simulink model "battery_pack_72v"  (R2020a)
settings: Solver=ode23t  StartTime=0.0  StopTime=5  RelTol=1e-3
libraries: fl_lib x1674, nesl_utility x2
(part 4 of 13)

== system battery_pack_72v/Battery_pack/Mod13/Cell2 ==
  Capacitor : fl_lib/Electrical/Electrical Elements/Capacitor  c=5000 F  r=1e-6 Ohm  g=0 1/Ohm  i_specify=off  i_priority=High  i=0 A  i_nominal_specify=off  i_nominal_unit=A  i_nominal_value=1  v_specify=off  v_priority=High  v=0 V  v_nominal_specify=off  v_nominal_unit=V  v_nominal_value=1  vc_specify=on  vc_priority=High  vc=0 V  vc_nominal_specify=off  vc_nominal_unit=V  vc_nominal_value=1
  DC Voltage Supply : fl_lib/Electrical/Electrical Sources/DC Voltage Source  v0=3.6 V
  Resistor1 : fl_lib/Electrical/Electrical Elements/Resistor  R=0.01 Ohm  i_specify=off  i_priority=High  i=0 A  i_nominal_specify=off  i_nominal_unit=A  i_nominal_value=1  v_specify=off  v_priority=High  v=0 V  v_nominal_specify=off  v_nominal_unit=V  v_nominal_value=1
  Resistor2 : fl_lib/Electrical/Electrical Elements/Resistor  R=0.005 Ohm  i_specify=off  i_priority=High  i=0 A  i_nominal_specify=off  i_nominal_unit=A  i_nominal_value=1  v_specify=off  v_priority=High  v=0 V  v_nominal_specify=off  v_nominal_unit=V  v_nominal_value=1
  + : PMIOPort  Side=Left
  - : PMIOPort  Port=2  Side=Right
  connections:
  DC Voltage Supply/LConn1 -- Resistor1/LConn1
  Capacitor/RConn1 -- +/RConn1 -- Resistor2/RConn1
  DC Voltage Supply/RConn1 -- -/RConn1
  Resistor1/RConn1 -- Capacitor/LConn1 -- Resistor2/LConn1

== system battery_pack_72v/Battery_pack/Mod13/Cell20 ==
  Capacitor : fl_lib/Electrical/Electrical Elements/Capacitor  c=5000 F  r=1e-6 Ohm  g=0 1/Ohm  i_specify=off  i_priority=High  i=0 A  i_nominal_specify=off  i_nominal_unit=A  i_nominal_value=1  v_specify=off  v_priority=High  v=0 V  v_nominal_specify=off  v_nominal_unit=V  v_nominal_value=1  vc_specify=on  vc_priority=High  vc=0 V  vc_nominal_specify=off  vc_nominal_unit=V  vc_nominal_value=1
  DC Voltage Supply : fl_lib/Electrical/Electrical Sources/DC Voltage Source  v0=3.6 V
  Resistor1 : fl_lib/Electrical/Electrical Elements/Resistor  R=0.01 Ohm  i_specify=off  i_priority=High  i=0 A  i_nominal_specify=off  i_nominal_unit=A  i_nominal_value=1  v_specify=off  v_priority=High  v=0 V  v_nominal_specify=off  v_nominal_unit=V  v_nominal_value=1
  Resistor2 : fl_lib/Electrical/Electrical Elements/Resistor  R=0.005 Ohm  i_specify=off  i_priority=High  i=0 A  i_nominal_specify=off  i_nominal_unit=A  i_nominal_value=1  v_specify=off  v_priority=High  v=0 V  v_nominal_specify=off  v_nominal_unit=V  v_nominal_value=1
  + : PMIOPort  Side=Left
  - : PMIOPort  Port=2  Side=Right
  connections:
  DC Voltage Supply/LConn1 -- Resistor1/LConn1
  Capacitor/RConn1 -- +/RConn1 -- Resistor2/RConn1
  DC Voltage Supply/RConn1 -- -/RConn1
  Resistor1/RConn1 -- Capacitor/LConn1 -- Resistor2/LConn1

== system battery_pack_72v/Battery_pack/Mod13/Cell21 ==
  Capacitor : fl_lib/Electrical/Electrical Elements/Capacitor  c=5000 F  r=1e-6 Ohm  g=0 1/Ohm  i_specify=off  i_priority=High  i=0 A  i_nominal_specify=off  i_nominal_unit=A  i_nominal_value=1  v_specify=off  v_priority=High  v=0 V  v_nominal_specify=off  v_nominal_unit=V  v_nominal_value=1  vc_specify=on  vc_priority=High  vc=0 V  vc_nominal_specify=off  vc_nominal_unit=V  vc_nominal_value=1
  DC Voltage Supply : fl_lib/Electrical/Electrical Sources/DC Voltage Source  v0=3.6 V
  Resistor1 : fl_lib/Electrical/Electrical Elements/Resistor  R=0.01 Ohm  i_specify=off  i_priority=High  i=0 A  i_nominal_specify=off  i_nominal_unit=A  i_nominal_value=1  v_specify=off  v_priority=High  v=0 V  v_nominal_specify=off  v_nominal_unit=V  v_nominal_value=1
  Resistor2 : fl_lib/Electrical/Electrical Elements/Resistor  R=0.005 Ohm  i_specify=off  i_priority=High  i=0 A  i_nominal_specify=off  i_nominal_unit=A  i_nominal_value=1  v_specify=off  v_priority=High  v=0 V  v_nominal_specify=off  v_nominal_unit=V  v_nominal_value=1
  + : PMIOPort  Side=Left
  - : PMIOPort  Port=2  Side=Right
  connections:
  Resistor2/LConn1 -- Capacitor/LConn1 -- Resistor1/RConn1
  DC Voltage Supply/RConn1 -- -/RConn1
  Resistor2/RConn1 -- +/RConn1 -- Capacitor/RConn1
  DC Voltage Supply/LConn1 -- Resistor1/LConn1

== system battery_pack_72v/Battery_pack/Mod13/Cell3 ==
  Capacitor : fl_lib/Electrical/Electrical Elements/Capacitor  c=5000 F  r=1e-6 Ohm  g=0 1/Ohm  i_specify=off  i_priority=High  i=0 A  i_nominal_specify=off  i_nominal_unit=A  i_nominal_value=1  v_specify=off  v_priority=High  v=0 V  v_nominal_specify=off  v_nominal_unit=V  v_nominal_value=1  vc_specify=on  vc_priority=High  vc=0 V  vc_nominal_specify=off  vc_nominal_unit=V  vc_nominal_value=1
  DC Voltage Supply : fl_lib/Electrical/Electrical Sources/DC Voltage Source  v0=3.6 V
  Resistor1 : fl_lib/Electrical/Electrical Elements/Resistor  R=0.01 Ohm  i_specify=off  i_priority=High  i=0 A  i_nominal_specify=off  i_nominal_unit=A  i_nominal_value=1  v_specify=off  v_priority=High  v=0 V  v_nominal_specify=off  v_nominal_unit=V  v_nominal_value=1
  Resistor2 : fl_lib/Electrical/Electrical Elements/Resistor  R=0.005 Ohm  i_specify=off  i_priority=High  i=0 A  i_nominal_specify=off  i_nominal_unit=A  i_nominal_value=1  v_specify=off  v_priority=High  v=0 V  v_nominal_specify=off  v_nominal_unit=V  v_nominal_value=1
  + : PMIOPort  Side=Left
  - : PMIOPort  Port=2  Side=Right
  connections:
  Resistor2/LConn1 -- Capacitor/LConn1 -- Resistor1/RConn1
  DC Voltage Supply/RConn1 -- -/RConn1
  Resistor2/RConn1 -- +/RConn1 -- Capacitor/RConn1
  DC Voltage Supply/LConn1 -- Resistor1/LConn1

== system battery_pack_72v/Battery_pack/Mod13/Cell4 ==
  Capacitor : fl_lib/Electrical/Electrical Elements/Capacitor  c=5000 F  r=1e-6 Ohm  g=0 1/Ohm  i_specify=off  i_priority=High  i=0 A  i_nominal_specify=off  i_nominal_unit=A  i_nominal_value=1  v_specify=off  v_priority=High  v=0 V  v_nominal_specify=off  v_nominal_unit=V  v_nominal_value=1  vc_specify=on  vc_priority=High  vc=0 V  vc_nominal_specify=off  vc_nominal_unit=V  vc_nominal_value=1
  DC Voltage Supply : fl_lib/Electrical/Electrical Sources/DC Voltage Source  v0=3.6 V
  Resistor1 : fl_lib/Electrical/Electrical Elements/Resistor  R=0.01 Ohm  i_specify=off  i_priority=High  i=0 A  i_nominal_specify=off  i_nominal_unit=A  i_nominal_value=1  v_specify=off  v_priority=High  v=0 V  v_nominal_specify=off  v_nominal_unit=V  v_nominal_value=1
  Resistor2 : fl_lib/Electrical/Electrical Elements/Resistor  R=0.005 Ohm  i_specify=off  i_priority=High  i=0 A  i_nominal_specify=off  i_nominal_unit=A  i_nominal_value=1  v_specify=off  v_priority=High  v=0 V  v_nominal_specify=off  v_nominal_unit=V  v_nominal_value=1
  + : PMIOPort  Side=Left
  - : PMIOPort  Port=2  Side=Right
  connections:
  DC Voltage Supply/LConn1 -- Resistor1/LConn1
  Capacitor/RConn1 -- +/RConn1 -- Resistor2/RConn1
  DC Voltage Supply/RConn1 -- -/RConn1
  Resistor1/RConn1 -- Capacitor/LConn1 -- Resistor2/LConn1

== system battery_pack_72v/Battery_pack/Mod13/Cell5 ==
  Capacitor : fl_lib/Electrical/Electrical Elements/Capacitor  c=5000 F  r=1e-6 Ohm  g=0 1/Ohm  i_specify=off  i_priority=High  i=0 A  i_nominal_specify=off  i_nominal_unit=A  i_nominal_value=1  v_specify=off  v_priority=High  v=0 V  v_nominal_specify=off  v_nominal_unit=V  v_nominal_value=1  vc_specify=on  vc_priority=High  vc=0 V  vc_nominal_specify=off  vc_nominal_unit=V  vc_nominal_value=1
  DC Voltage Supply : fl_lib/Electrical/Electrical Sources/DC Voltage Source  v0=3.6 V
  Resistor1 : fl_lib/Electrical/Electrical Elements/Resistor  R=0.01 Ohm  i_specify=off  i_priority=High  i=0 A  i_nominal_specify=off  i_nominal_unit=A  i_nominal_value=1  v_specify=off  v_priority=High  v=0 V  v_nominal_specify=off  v_nominal_unit=V  v_nominal_value=1
  Resistor2 : fl_lib/Electrical/Electrical Elements/Resistor  R=0.005 Ohm  i_specify=off  i_priority=High  i=0 A  i_nominal_specify=off  i_nominal_unit=A  i_nominal_value=1  v_specify=off  v_priority=High  v=0 V  v_nominal_specify=off  v_nominal_unit=V  v_nominal_value=1
  + : PMIOPort  Side=Left
  - : PMIOPort  Port=2  Side=Right
  connections:
  Resistor2/LConn1 -- Capacitor/LConn1 -- Resistor1/RConn1
  DC Voltage Supply/RConn1 -- -/RConn1
  Resistor2/RConn1 -- +/RConn1 -- Capacitor/RConn1
  DC Voltage Supply/LConn1 -- Resistor1/LConn1

== system battery_pack_72v/Battery_pack/Mod13/Cell6 ==
  Capacitor : fl_lib/Electrical/Electrical Elements/Capacitor  c=5000 F  r=1e-6 Ohm  g=0 1/Ohm  i_specify=off  i_priority=High  i=0 A  i_nominal_specify=off  i_nominal_unit=A  i_nominal_value=1  v_specify=off  v_priority=High  v=0 V  v_nominal_specify=off  v_nominal_unit=V  v_nominal_value=1  vc_specify=on  vc_priority=High  vc=0 V  vc_nominal_specify=off  vc_nominal_unit=V  vc_nominal_value=1
  DC Voltage Supply : fl_lib/Electrical/Electrical Sources/DC Voltage Source  v0=3.6 V
  Resistor1 : fl_lib/Electrical/Electrical Elements/Resistor  R=0.01 Ohm  i_specify=off  i_priority=High  i=0 A  i_nominal_specify=off  i_nominal_unit=A  i_nominal_value=1  v_specify=off  v_priority=High  v=0 V  v_nominal_specify=off  v_nominal_unit=V  v_nominal_value=1
  Resistor2 : fl_lib/Electrical/Electrical Elements/Resistor  R=0.005 Ohm  i_specify=off  i_priority=High  i=0 A  i_nominal_specify=off  i_nominal_unit=A  i_nominal_value=1  v_specify=off  v_priority=High  v=0 V  v_nominal_specify=off  v_nominal_unit=V  v_nominal_value=1
  + : PMIOPort  Side=Left
  - : PMIOPort  Port=2  Side=Right
  connections:
  DC Voltage Supply/LConn1 -- Resistor1/LConn1
  Capacitor/RConn1 -- +/RConn1 -- Resistor2/RConn1
  DC Voltage Supply/RConn1 -- -/RConn1
  Resistor1/RConn1 -- Capacitor/LConn1 -- Resistor2/LConn1

== system battery_pack_72v/Battery_pack/Mod13/Cell7 ==
  Capacitor : fl_lib/Electrical/Electrical Elements/Capacitor  c=5000 F  r=1e-6 Ohm  g=0 1/Ohm  i_specify=off  i_priority=High  i=0 A  i_nominal_specify=off  i_nominal_unit=A  i_nominal_value=1  v_specify=off  v_priority=High  v=0 V  v_nominal_specify=off  v_nominal_unit=V  v_nominal_value=1  vc_specify=on  vc_priority=High  vc=0 V  vc_nominal_specify=off  vc_nominal_unit=V  vc_nominal_value=1
  DC Voltage Supply : fl_lib/Electrical/Electrical Sources/DC Voltage Source  v0=3.6 V
  Resistor1 : fl_lib/Electrical/Electrical Elements/Resistor  R=0.01 Ohm  i_specify=off  i_priority=High  i=0 A  i_nominal_specify=off  i_nominal_unit=A  i_nominal_value=1  v_specify=off  v_priority=High  v=0 V  v_nominal_specify=off  v_nominal_unit=V  v_nominal_value=1
  Resistor2 : fl_lib/Electrical/Electrical Elements/Resistor  R=0.005 Ohm  i_specify=off  i_priority=High  i=0 A  i_nominal_specify=off  i_nominal_unit=A  i_nominal_value=1  v_specify=off  v_priority=High  v=0 V  v_nominal_specify=off  v_nominal_unit=V  v_nominal_value=1
  + : PMIOPort  Side=Left
  - : PMIOPort  Port=2  Side=Right
  connections:
  Resistor2/LConn1 -- Capacitor/LConn1 -- Resistor1/RConn1
  DC Voltage Supply/RConn1 -- -/RConn1
  Resistor2/RConn1 -- +/RConn1 -- Capacitor/RConn1
  DC Voltage Supply/LConn1 -- Resistor1/LConn1

== system battery_pack_72v/Battery_pack/Mod13/Cell8 ==
  Capacitor : fl_lib/Electrical/Electrical Elements/Capacitor  c=5000 F  r=1e-6 Ohm  g=0 1/Ohm  i_specify=off  i_priority=High  i=0 A  i_nominal_specify=off  i_nominal_unit=A  i_nominal_value=1  v_specify=off  v_priority=High  v=0 V  v_nominal_specify=off  v_nominal_unit=V  v_nominal_value=1  vc_specify=on  vc_priority=High  vc=0 V  vc_nominal_specify=off  vc_nominal_unit=V  vc_nominal_value=1
  DC Voltage Supply : fl_lib/Electrical/Electrical Sources/DC Voltage Source  v0=3.6 V
  Resistor1 : fl_lib/Electrical/Electrical Elements/Resistor  R=0.01 Ohm  i_specify=off  i_priority=High  i=0 A  i_nominal_specify=off  i_nominal_unit=A  i_nominal_value=1  v_specify=off  v_priority=High  v=0 V  v_nominal_specify=off  v_nominal_unit=V  v_nominal_value=1
  Resistor2 : fl_lib/Electrical/Electrical Elements/Resistor  R=0.005 Ohm  i_specify=off  i_priority=High  i=0 A  i_nominal_specify=off  i_nominal_unit=A  i_nominal_value=1  v_specify=off  v_priority=High  v=0 V  v_nominal_specify=off  v_nominal_unit=V  v_nominal_value=1
  + : PMIOPort  Side=Left
  - : PMIOPort  Port=2  Side=Right
  connections:
  DC Voltage Supply/LConn1 -- Resistor1/LConn1
  Capacitor/RConn1 -- +/RConn1 -- Resistor2/RConn1
  DC Voltage Supply/RConn1 -- -/RConn1
  Resistor1/RConn1 -- Capacitor/LConn1 -- Resistor2/LConn1

== system battery_pack_72v/Battery_pack/Mod13/Cell9 ==
  Capacitor : fl_lib/Electrical/Electrical Elements/Capacitor  c=5000 F  r=1e-6 Ohm  g=0 1/Ohm  i_specify=off  i_priority=High  i=0 A  i_nominal_specify=off  i_nominal_unit=A  i_nominal_value=1  v_specify=off  v_priority=High  v=0 V  v_nominal_specify=off  v_nominal_unit=V  v_nominal_value=1  vc_specify=on  vc_priority=High  vc=0 V  vc_nominal_specify=off  vc_nominal_unit=V  vc_nominal_value=1
  DC Voltage Supply : fl_lib/Electrical/Electrical Sources/DC Voltage Source  v0=3.6 V
  Resistor1 : fl_lib/Electrical/Electrical Elements/Resistor  R=0.01 Ohm  i_specify=off  i_priority=High  i=0 A  i_nominal_specify=off  i_nominal_unit=A  i_nominal_value=1  v_specify=off  v_priority=High  v=0 V  v_nominal_specify=off  v_nominal_unit=V  v_nominal_value=1
  Resistor2 : fl_lib/Electrical/Electrical Elements/Resistor  R=0.005 Ohm  i_specify=off  i_priority=High  i=0 A  i_nominal_specify=off  i_nominal_unit=A  i_nominal_value=1  v_specify=off  v_priority=High  v=0 V  v_nominal_specify=off  v_nominal_unit=V  v_nominal_value=1
  + : PMIOPort  Side=Left
  - : PMIOPort  Port=2  Side=Right
  connections:
  Resistor2/LConn1 -- Capacitor/LConn1 -- Resistor1/RConn1
  DC Voltage Supply/RConn1 -- -/RConn1
  Resistor2/RConn1 -- +/RConn1 -- Capacitor/RConn1
  DC Voltage Supply/LConn1 -- Resistor1/LConn1

== system battery_pack_72v/Battery_pack/Mod14/Cell1 ==
  Capacitor : fl_lib/Electrical/Electrical Elements/Capacitor  c=5000 F  r=1e-6 Ohm  g=0 1/Ohm  i_specify=off  i_priority=High  i=0 A  i_nominal_specify=off  i_nominal_unit=A  i_nominal_value=1  v_specify=off  v_priority=High  v=0 V  v_nominal_specify=off  v_nominal_unit=V  v_nominal_value=1  vc_specify=on  vc_priority=High  vc=0 V  vc_nominal_specify=off  vc_nominal_unit=V  vc_nominal_value=1
  DC Voltage Supply : fl_lib/Electrical/Electrical Sources/DC Voltage Source  v0=3.6 V
  Resistor1 : fl_lib/Electrical/Electrical Elements/Resistor  R=0.01 Ohm  i_specify=off  i_priority=High  i=0 A  i_nominal_specify=off  i_nominal_unit=A  i_nominal_value=1  v_specify=off  v_priority=High  v=0 V  v_nominal_specify=off  v_nominal_unit=V  v_nominal_value=1
  Resistor2 : fl_lib/Electrical/Electrical Elements/Resistor  R=0.005 Ohm  i_specify=off  i_priority=High  i=0 A  i_nominal_specify=off  i_nominal_unit=A  i_nominal_value=1  v_specify=off  v_priority=High  v=0 V  v_nominal_specify=off  v_nominal_unit=V  v_nominal_value=1
  + : PMIOPort  Side=Left
  - : PMIOPort  Port=2  Side=Right
  connections:
  DC Voltage Supply/LConn1 -- Resistor1/LConn1
  Capacitor/RConn1 -- +/RConn1 -- Resistor2/RConn1
  DC Voltage Supply/RConn1 -- -/RConn1
  Resistor1/RConn1 -- Capacitor/LConn1 -- Resistor2/LConn1

== system battery_pack_72v/Battery_pack/Mod14/Cell10 ==
  Capacitor : fl_lib/Electrical/Electrical Elements/Capacitor  c=5000 F  r=1e-6 Ohm  g=0 1/Ohm  i_specify=off  i_priority=High  i=0 A  i_nominal_specify=off  i_nominal_unit=A  i_nominal_value=1  v_specify=off  v_priority=High  v=0 V  v_nominal_specify=off  v_nominal_unit=V  v_nominal_value=1  vc_specify=on  vc_priority=High  vc=0 V  vc_nominal_specify=off  vc_nominal_unit=V  vc_nominal_value=1
  DC Voltage Supply : fl_lib/Electrical/Electrical Sources/DC Voltage Source  v0=3.6 V
  Resistor1 : fl_lib/Electrical/Electrical Elements/Resistor  R=0.01 Ohm  i_specify=off  i_priority=High  i=0 A  i_nominal_specify=off  i_nominal_unit=A  i_nominal_value=1  v_specify=off  v_priority=High  v=0 V  v_nominal_specify=off  v_nominal_unit=V  v_nominal_value=1
  Resistor2 : fl_lib/Electrical/Electrical Elements/Resistor  R=0.005 Ohm  i_specify=off  i_priority=High  i=0 A  i_nominal_specify=off  i_nominal_unit=A  i_nominal_value=1  v_specify=off  v_priority=High  v=0 V  v_nominal_specify=off  v_nominal_unit=V  v_nominal_value=1
  + : PMIOPort  Side=Left
  - : PMIOPort  Port=2  Side=Right
  connections:
  Resistor2/LConn1 -- Capacitor/LConn1 -- Resistor1/RConn1
  DC Voltage Supply/RConn1 -- -/RConn1
  Resistor2/RConn1 -- +/RConn1 -- Capacitor/RConn1
  DC Voltage Supply/LConn1 -- Resistor1/LConn1

== system battery_pack_72v/Battery_pack/Mod14/Cell11 ==
  Capacitor : fl_lib/Electrical/Electrical Elements/Capacitor  c=5000 F  r=1e-6 Ohm  g=0 1/Ohm  i_specify=off  i_priority=High  i=0 A  i_nominal_specify=off  i_nominal_unit=A  i_nominal_value=1  v_specify=off  v_priority=High  v=0 V  v_nominal_specify=off  v_nominal_unit=V  v_nominal_value=1  vc_specify=on  vc_priority=High  vc=0 V  vc_nominal_specify=off  vc_nominal_unit=V  vc_nominal_value=1
  DC Voltage Supply : fl_lib/Electrical/Electrical Sources/DC Voltage Source  v0=3.6 V
  Resistor1 : fl_lib/Electrical/Electrical Elements/Resistor  R=0.01 Ohm  i_specify=off  i_priority=High  i=0 A  i_nominal_specify=off  i_nominal_unit=A  i_nominal_value=1  v_specify=off  v_priority=High  v=0 V  v_nominal_specify=off  v_nominal_unit=V  v_nominal_value=1
  Resistor2 : fl_lib/Electrical/Electrical Elements/Resistor  R=0.005 Ohm  i_specify=off  i_priority=High  i=0 A  i_nominal_specify=off  i_nominal_unit=A  i_nominal_value=1  v_specify=off  v_priority=High  v=0 V  v_nominal_specify=off  v_nominal_unit=V  v_nominal_value=1
  + : PMIOPort  Side=Left
  - : PMIOPort  Port=2  Side=Right
  connections:
  DC Voltage Supply/LConn1 -- Resistor1/LConn1
  Capacitor/RConn1 -- +/RConn1 -- Resistor2/RConn1
  DC Voltage Supply/RConn1 -- -/RConn1
  Resistor1/RConn1 -- Capacitor/LConn1 -- Resistor2/LConn1

== system battery_pack_72v/Battery_pack/Mod14/Cell12 ==
  Capacitor : fl_lib/Electrical/Electrical Elements/Capacitor  c=5000 F  r=1e-6 Ohm  g=0 1/Ohm  i_specify=off  i_priority=High  i=0 A  i_nominal_specify=off  i_nominal_unit=A  i_nominal_value=1  v_specify=off  v_priority=High  v=0 V  v_nominal_specify=off  v_nominal_unit=V  v_nominal_value=1  vc_specify=on  vc_priority=High  vc=0 V  vc_nominal_specify=off  vc_nominal_unit=V  vc_nominal_value=1
  DC Voltage Supply : fl_lib/Electrical/Electrical Sources/DC Voltage Source  v0=3.6 V
  Resistor1 : fl_lib/Electrical/Electrical Elements/Resistor  R=0.01 Ohm  i_specify=off  i_priority=High  i=0 A  i_nominal_specify=off  i_nominal_unit=A  i_nominal_value=1  v_specify=off  v_priority=High  v=0 V  v_nominal_specify=off  v_nominal_unit=V  v_nominal_value=1
  Resistor2 : fl_lib/Electrical/Electrical Elements/Resistor  R=0.005 Ohm  i_specify=off  i_priority=High  i=0 A  i_nominal_specify=off  i_nominal_unit=A  i_nominal_value=1  v_specify=off  v_priority=High  v=0 V  v_nominal_specify=off  v_nominal_unit=V  v_nominal_value=1
  + : PMIOPort  Side=Left
  - : PMIOPort  Port=2  Side=Right
  connections:
  Resistor2/LConn1 -- Capacitor/LConn1 -- Resistor1/RConn1
  DC Voltage Supply/RConn1 -- -/RConn1
  Resistor2/RConn1 -- +/RConn1 -- Capacitor/RConn1
  DC Voltage Supply/LConn1 -- Resistor1/LConn1

== system battery_pack_72v/Battery_pack/Mod14/Cell15 ==
  Capacitor : fl_lib/Electrical/Electrical Elements/Capacitor  c=5000 F  r=1e-6 Ohm  g=0 1/Ohm  i_specify=off  i_priority=High  i=0 A  i_nominal_specify=off  i_nominal_unit=A  i_nominal_value=1  v_specify=off  v_priority=High  v=0 V  v_nominal_specify=off  v_nominal_unit=V  v_nominal_value=1  vc_specify=on  vc_priority=High  vc=0 V  vc_nominal_specify=off  vc_nominal_unit=V  vc_nominal_value=1
  DC Voltage Supply : fl_lib/Electrical/Electrical Sources/DC Voltage Source  v0=3.6 V
  Resistor1 : fl_lib/Electrical/Electrical Elements/Resistor  R=0.01 Ohm  i_specify=off  i_priority=High  i=0 A  i_nominal_specify=off  i_nominal_unit=A  i_nominal_value=1  v_specify=off  v_priority=High  v=0 V  v_nominal_specify=off  v_nominal_unit=V  v_nominal_value=1
  Resistor2 : fl_lib/Electrical/Electrical Elements/Resistor  R=0.005 Ohm  i_specify=off  i_priority=High  i=0 A  i_nominal_specify=off  i_nominal_unit=A  i_nominal_value=1  v_specify=off  v_priority=High  v=0 V  v_nominal_specify=off  v_nominal_unit=V  v_nominal_value=1
  + : PMIOPort  Side=Left
  - : PMIOPort  Port=2  Side=Right
  connections:
  DC Voltage Supply/LConn1 -- Resistor1/LConn1
  Capacitor/RConn1 -- +/RConn1 -- Resistor2/RConn1
  DC Voltage Supply/RConn1 -- -/RConn1
  Resistor1/RConn1 -- Capacitor/LConn1 -- Resistor2/LConn1

== system battery_pack_72v/Battery_pack/Mod14/Cell16 ==
  Capacitor : fl_lib/Electrical/Electrical Elements/Capacitor  c=5000 F  r=1e-6 Ohm  g=0 1/Ohm  i_specify=off  i_priority=High  i=0 A  i_nominal_specify=off  i_nominal_unit=A  i_nominal_value=1  v_specify=off  v_priority=High  v=0 V  v_nominal_specify=off  v_nominal_unit=V  v_nominal_value=1  vc_specify=on  vc_priority=High  vc=0 V  vc_nominal_specify=off  vc_nominal_unit=V  vc_nominal_value=1
  DC Voltage Supply : fl_lib/Electrical/Electrical Sources/DC Voltage Source  v0=3.6 V
  Resistor1 : fl_lib/Electrical/Electrical Elements/Resistor  R=0.01 Ohm  i_specify=off  i_priority=High  i=0 A  i_nominal_specify=off  i_nominal_unit=A  i_nominal_value=1  v_specify=off  v_priority=High  v=0 V  v_nominal_specify=off  v_nominal_unit=V  v_nominal_value=1
  Resistor2 : fl_lib/Electrical/Electrical Elements/Resistor  R=0.005 Ohm  i_specify=off  i_priority=High  i=0 A  i_nominal_specify=off  i_nominal_unit=A  i_nominal_value=1  v_specify=off  v_priority=High  v=0 V  v_nominal_specify=off  v_nominal_unit=V  v_nominal_value=1
  + : PMIOPort  Side=Left
  - : PMIOPort  Port=2  Side=Right
  connections:
  Resistor2/LConn1 -- Capacitor/LConn1 -- Resistor1/RConn1
  DC Voltage Supply/RConn1 -- -/RConn1
  Resistor2/RConn1 -- +/RConn1 -- Capacitor/RConn1
  DC Voltage Supply/LConn1 -- Resistor1/LConn1

== system battery_pack_72v/Battery_pack/Mod14/Cell17 ==
  Capacitor : fl_lib/Electrical/Electrical Elements/Capacitor  c=5000 F  r=1e-6 Ohm  g=0 1/Ohm  i_specify=off  i_priority=High  i=0 A  i_nominal_specify=off  i_nominal_unit=A  i_nominal_value=1  v_specify=off  v_priority=High  v=0 V  v_nominal_specify=off  v_nominal_unit=V  v_nominal_value=1  vc_specify=on  vc_priority=High  vc=0 V  vc_nominal_specify=off  vc_nominal_unit=V  vc_nominal_value=1
  DC Voltage Supply : fl_lib/Electrical/Electrical Sources/DC Voltage Source  v0=3.6 V
  Resistor1 : fl_lib/Electrical/Electrical Elements/Resistor  R=0.01 Ohm  i_specify=off  i_priority=High  i=0 A  i_nominal_specify=off  i_nominal_unit=A  i_nominal_value=1  v_specify=off  v_priority=High  v=0 V  v_nominal_specify=off  v_nominal_unit=V  v_nominal_value=1
  Resistor2 : fl_lib/Electrical/Electrical Elements/Resistor  R=0.005 Ohm  i_specify=off  i_priority=High  i=0 A  i_nominal_specify=off  i_nominal_unit=A  i_nominal_value=1  v_specify=off  v_priority=High  v=0 V  v_nominal_specify=off  v_nominal_unit=V  v_nominal_value=1
  + : PMIOPort  Side=Left
  - : PMIOPort  Port=2  Side=Right
  connections:
  DC Voltage Supply/LConn1 -- Resistor1/LConn1
  Capacitor/RConn1 -- +/RConn1 -- Resistor2/RConn1
  DC Voltage Supply/RConn1 -- -/RConn1
  Resistor1/RConn1 -- Capacitor/LConn1 -- Resistor2/LConn1

== system battery_pack_72v/Battery_pack/Mod14/Cell18 ==
  Capacitor : fl_lib/Electrical/Electrical Elements/Capacitor  c=5000 F  r=1e-6 Ohm  g=0 1/Ohm  i_specify=off  i_priority=High  i=0 A  i_nominal_specify=off  i_nominal_unit=A  i_nominal_value=1  v_specify=off  v_priority=High  v=0 V  v_nominal_specify=off  v_nominal_unit=V  v_nominal_value=1  vc_specify=on  vc_priority=High  vc=0 V  vc_nominal_specify=off  vc_nominal_unit=V  vc_nominal_value=1
  DC Voltage Supply : fl_lib/Electrical/Electrical Sources/DC Voltage Source  v0=3.6 V
  Resistor1 : fl_lib/Electrical/Electrical Elements/Resistor  R=0.01 Ohm  i_specify=off  i_priority=High  i=0 A  i_nominal_specify=off  i_nominal_unit=A  i_nominal_value=1  v_specify=off  v_priority=High  v=0 V  v_nominal_specify=off  v_nominal_unit=V  v_nominal_value=1
  Resistor2 : fl_lib/Electrical/Electrical Elements/Resistor  R=0.005 Ohm  i_specify=off  i_priority=High  i=0 A  i_nominal_specify=off  i_nominal_unit=A  i_nominal_value=1  v_specify=off  v_priority=High  v=0 V  v_nominal_specify=off  v_nominal_unit=V  v_nominal_value=1
  + : PMIOPort  Side=Left
  - : PMIOPort  Port=2  Side=Right
  connections:
  Resistor2/LConn1 -- Capacitor/LConn1 -- Resistor1/RConn1
  DC Voltage Supply/RConn1 -- -/RConn1
  Resistor2/RConn1 -- +/RConn1 -- Capacitor/RConn1
  DC Voltage Supply/LConn1 -- Resistor1/LConn1

== system battery_pack_72v/Battery_pack/Mod14/Cell19 ==
  Capacitor : fl_lib/Electrical/Electrical Elements/Capacitor  c=5000 F  r=1e-6 Ohm  g=0 1/Ohm  i_specify=off  i_priority=High  i=0 A  i_nominal_specify=off  i_nominal_unit=A  i_nominal_value=1  v_specify=off  v_priority=High  v=0 V  v_nominal_specify=off  v_nominal_unit=V  v_nominal_value=1  vc_specify=on  vc_priority=High  vc=0 V  vc_nominal_specify=off  vc_nominal_unit=V  vc_nominal_value=1
  DC Voltage Supply : fl_lib/Electrical/Electrical Sources/DC Voltage Source  v0=3.6 V
  Resistor1 : fl_lib/Electrical/Electrical Elements/Resistor  R=0.01 Ohm  i_specify=off  i_priority=High  i=0 A  i_nominal_specify=off  i_nominal_unit=A  i_nominal_value=1  v_specify=off  v_priority=High  v=0 V  v_nominal_specify=off  v_nominal_unit=V  v_nominal_value=1
  Resistor2 : fl_lib/Electrical/Electrical Elements/Resistor  R=0.005 Ohm  i_specify=off  i_priority=High  i=0 A  i_nominal_specify=off  i_nominal_unit=A  i_nominal_value=1  v_specify=off  v_priority=High  v=0 V  v_nominal_specify=off  v_nominal_unit=V  v_nominal_value=1
  + : PMIOPort  Side=Left
  - : PMIOPort  Port=2  Side=Right
  connections:
  DC Voltage Supply/LConn1 -- Resistor1/LConn1
  Capacitor/RConn1 -- +/RConn1 -- Resistor2/RConn1
  DC Voltage Supply/RConn1 -- -/RConn1
  Resistor1/RConn1 -- Capacitor/LConn1 -- Resistor2/LConn1

== system battery_pack_72v/Battery_pack/Mod14/Cell2 ==
  Capacitor : fl_lib/Electrical/Electrical Elements/Capacitor  c=5000 F  r=1e-6 Ohm  g=0 1/Ohm  i_specify=off  i_priority=High  i=0 A  i_nominal_specify=off  i_nominal_unit=A  i_nominal_value=1  v_specify=off  v_priority=High  v=0 V  v_nominal_specify=off  v_nominal_unit=V  v_nominal_value=1  vc_specify=on  vc_priority=High  vc=0 V  vc_nominal_specify=off  vc_nominal_unit=V  vc_nominal_value=1
  DC Voltage Supply : fl_lib/Electrical/Electrical Sources/DC Voltage Source  v0=3.6 V
  Resistor1 : fl_lib/Electrical/Electrical Elements/Resistor  R=0.01 Ohm  i_specify=off  i_priority=High  i=0 A  i_nominal_specify=off  i_nominal_unit=A  i_nominal_value=1  v_specify=off  v_priority=High  v=0 V  v_nominal_specify=off  v_nominal_unit=V  v_nominal_value=1
  Resistor2 : fl_lib/Electrical/Electrical Elements/Resistor  R=0.005 Ohm  i_specify=off  i_priority=High  i=0 A  i_nominal_specify=off  i_nominal_unit=A  i_nominal_value=1  v_specify=off  v_priority=High  v=0 V  v_nominal_specify=off  v_nominal_unit=V  v_nominal_value=1
  + : PMIOPort  Side=Left
  - : PMIOPort  Port=2  Side=Right
  connections:
  Resistor2/LConn1 -- Capacitor/LConn1 -- Resistor1/RConn1
  DC Voltage Supply/RConn1 -- -/RConn1
  Resistor2/RConn1 -- +/RConn1 -- Capacitor/RConn1
  DC Voltage Supply/LConn1 -- Resistor1/LConn1

== system battery_pack_72v/Battery_pack/Mod14/Cell20 ==
  Capacitor : fl_lib/Electrical/Electrical Elements/Capacitor  c=5000 F  r=1e-6 Ohm  g=0 1/Ohm  i_specify=off  i_priority=High  i=0 A  i_nominal_specify=off  i_nominal_unit=A  i_nominal_value=1  v_specify=off  v_priority=High  v=0 V  v_nominal_specify=off  v_nominal_unit=V  v_nominal_value=1  vc_specify=on  vc_priority=High  vc=0 V  vc_nominal_specify=off  vc_nominal_unit=V  vc_nominal_value=1
  DC Voltage Supply : fl_lib/Electrical/Electrical Sources/DC Voltage Source  v0=3.6 V
  Resistor1 : fl_lib/Electrical/Electrical Elements/Resistor  R=0.01 Ohm  i_specify=off  i_priority=High  i=0 A  i_nominal_specify=off  i_nominal_unit=A  i_nominal_value=1  v_specify=off  v_priority=High  v=0 V  v_nominal_specify=off  v_nominal_unit=V  v_nominal_value=1
  Resistor2 : fl_lib/Electrical/Electrical Elements/Resistor  R=0.005 Ohm  i_specify=off  i_priority=High  i=0 A  i_nominal_specify=off  i_nominal_unit=A  i_nominal_value=1  v_specify=off  v_priority=High  v=0 V  v_nominal_specify=off  v_nominal_unit=V  v_nominal_value=1
  + : PMIOPort  Side=Left
  - : PMIOPort  Port=2  Side=Right
  connections:
  Resistor2/LConn1 -- Capacitor/LConn1 -- Resistor1/RConn1
  DC Voltage Supply/RConn1 -- -/RConn1
  Resistor2/RConn1 -- +/RConn1 -- Capacitor/RConn1
  DC Voltage Supply/LConn1 -- Resistor1/LConn1

== system battery_pack_72v/Battery_pack/Mod14/Cell21 ==
  Capacitor : fl_lib/Electrical/Electrical Elements/Capacitor  c=5000 F  r=1e-6 Ohm  g=0 1/Ohm  i_specify=off  i_priority=High  i=0 A  i_nominal_specify=off  i_nominal_unit=A  i_nominal_value=1  v_specify=off  v_priority=High  v=0 V  v_nominal_specify=off  v_nominal_unit=V  v_nominal_value=1  vc_specify=on  vc_priority=High  vc=0 V  vc_nominal_specify=off  vc_nominal_unit=V  vc_nominal_value=1
  DC Voltage Supply : fl_lib/Electrical/Electrical Sources/DC Voltage Source  v0=3.6 V
  Resistor1 : fl_lib/Electrical/Electrical Elements/Resistor  R=0.01 Ohm  i_specify=off  i_priority=High  i=0 A  i_nominal_specify=off  i_nominal_unit=A  i_nominal_value=1  v_specify=off  v_priority=High  v=0 V  v_nominal_specify=off  v_nominal_unit=V  v_nominal_value=1
  Resistor2 : fl_lib/Electrical/Electrical Elements/Resistor  R=0.005 Ohm  i_specify=off  i_priority=High  i=0 A  i_nominal_specify=off  i_nominal_unit=A  i_nominal_value=1  v_specify=off  v_priority=High  v=0 V  v_nominal_specify=off  v_nominal_unit=V  v_nominal_value=1
  + : PMIOPort  Side=Left
  - : PMIOPort  Port=2  Side=Right
  connections:
  DC Voltage Supply/LConn1 -- Resistor1/LConn1
  Capacitor/RConn1 -- +/RConn1 -- Resistor2/RConn1
  DC Voltage Supply/RConn1 -- -/RConn1
  Resistor1/RConn1 -- Capacitor/LConn1 -- Resistor2/LConn1

== system battery_pack_72v/Battery_pack/Mod14/Cell3 ==
  Capacitor : fl_lib/Electrical/Electrical Elements/Capacitor  c=5000 F  r=1e-6 Ohm  g=0 1/Ohm  i_specify=off  i_priority=High  i=0 A  i_nominal_specify=off  i_nominal_unit=A  i_nominal_value=1  v_specify=off  v_priority=High  v=0 V  v_nominal_specify=off  v_nominal_unit=V  v_nominal_value=1  vc_specify=on  vc_priority=High  vc=0 V  vc_nominal_specify=off  vc_nominal_unit=V  vc_nominal_value=1
  DC Voltage Supply : fl_lib/Electrical/Electrical Sources/DC Voltage Source  v0=3.6 V
  Resistor1 : fl_lib/Electrical/Electrical Elements/Resistor  R=0.01 Ohm  i_specify=off  i_priority=High  i=0 A  i_nominal_specify=off  i_nominal_unit=A  i_nominal_value=1  v_specify=off  v_priority=High  v=0 V  v_nominal_specify=off  v_nominal_unit=V  v_nominal_value=1
  Resistor2 : fl_lib/Electrical/Electrical Elements/Resistor  R=0.005 Ohm  i_specify=off  i_priority=High  i=0 A  i_nominal_specify=off  i_nominal_unit=A  i_nominal_value=1  v_specify=off  v_priority=High  v=0 V  v_nominal_specify=off  v_nominal_unit=V  v_nominal_value=1
  + : PMIOPort  Side=Left
  - : PMIOPort  Port=2  Side=Right
  connections:
  DC Voltage Supply/LConn1 -- Resistor1/LConn1
  Capacitor/RConn1 -- +/RConn1 -- Resistor2/RConn1
  DC Voltage Supply/RConn1 -- -/RConn1
  Resistor1/RConn1 -- Capacitor/LConn1 -- Resistor2/LConn1

== system battery_pack_72v/Battery_pack/Mod14/Cell4 ==
  Capacitor : fl_lib/Electrical/Electrical Elements/Capacitor  c=5000 F  r=1e-6 Ohm  g=0 1/Ohm  i_specify=off  i_priority=High  i=0 A  i_nominal_specify=off  i_nominal_unit=A  i_nominal_value=1  v_specify=off  v_priority=High  v=0 V  v_nominal_specify=off  v_nominal_unit=V  v_nominal_value=1  vc_specify=on  vc_priority=High  vc=0 V  vc_nominal_specify=off  vc_nominal_unit=V  vc_nominal_value=1
  DC Voltage Supply : fl_lib/Electrical/Electrical Sources/DC Voltage Source  v0=3.6 V
  Resistor1 : fl_lib/Electrical/Electrical Elements/Resistor  R=0.01 Ohm  i_specify=off  i_priority=High  i=0 A  i_nominal_specify=off  i_nominal_unit=A  i_nominal_value=1  v_specify=off  v_priority=High  v=0 V  v_nominal_specify=off  v_nominal_unit=V  v_nominal_value=1
  Resistor2 : fl_lib/Electrical/Electrical Elements/Resistor  R=0.005 Ohm  i_specify=off  i_priority=High  i=0 A  i_nominal_specify=off  i_nominal_unit=A  i_nominal_value=1  v_specify=off  v_priority=High  v=0 V  v_nominal_specify=off  v_nominal_unit=V  v_nominal_value=1
  + : PMIOPort  Side=Left
  - : PMIOPort  Port=2  Side=Right
  connections:
  Resistor2/LConn1 -- Capacitor/LConn1 -- Resistor1/RConn1
  DC Voltage Supply/RConn1 -- -/RConn1
  Resistor2/RConn1 -- +/RConn1 -- Capacitor/RConn1
  DC Voltage Supply/LConn1 -- Resistor1/LConn1

== system battery_pack_72v/Battery_pack/Mod14/Cell5 ==
  Capacitor : fl_lib/Electrical/Electrical Elements/Capacitor  c=5000 F  r=1e-6 Ohm  g=0 1/Ohm  i_specify=off  i_priority=High  i=0 A  i_nominal_specify=off  i_nominal_unit=A  i_nominal_value=1  v_specify=off  v_priority=High  v=0 V  v_nominal_specify=off  v_nominal_unit=V  v_nominal_value=1  vc_specify=on  vc_priority=High  vc=0 V  vc_nominal_specify=off  vc_nominal_unit=V  vc_nominal_value=1
  DC Voltage Supply : fl_lib/Electrical/Electrical Sources/DC Voltage Source  v0=3.6 V
  Resistor1 : fl_lib/Electrical/Electrical Elements/Resistor  R=0.01 Ohm  i_specify=off  i_priority=High  i=0 A  i_nominal_specify=off  i_nominal_unit=A  i_nominal_value=1  v_specify=off  v_priority=High  v=0 V  v_nominal_specify=off  v_nominal_unit=V  v_nominal_value=1
  Resistor2 : fl_lib/Electrical/Electrical Elements/Resistor  R=0.005 Ohm  i_specify=off  i_priority=High  i=0 A  i_nominal_specify=off  i_nominal_unit=A  i_nominal_value=1  v_specify=off  v_priority=High  v=0 V  v_nominal_specify=off  v_nominal_unit=V  v_nominal_value=1
  + : PMIOPort  Side=Left
  - : PMIOPort  Port=2  Side=Right
  connections:
  DC Voltage Supply/LConn1 -- Resistor1/LConn1
  Capacitor/RConn1 -- +/RConn1 -- Resistor2/RConn1
  DC Voltage Supply/RConn1 -- -/RConn1
  Resistor1/RConn1 -- Capacitor/LConn1 -- Resistor2/LConn1

== system battery_pack_72v/Battery_pack/Mod14/Cell6 ==
  Capacitor : fl_lib/Electrical/Electrical Elements/Capacitor  c=5000 F  r=1e-6 Ohm  g=0 1/Ohm  i_specify=off  i_priority=High  i=0 A  i_nominal_specify=off  i_nominal_unit=A  i_nominal_value=1  v_specify=off  v_priority=High  v=0 V  v_nominal_specify=off  v_nominal_unit=V  v_nominal_value=1  vc_specify=on  vc_priority=High  vc=0 V  vc_nominal_specify=off  vc_nominal_unit=V  vc_nominal_value=1
  DC Voltage Supply : fl_lib/Electrical/Electrical Sources/DC Voltage Source  v0=3.6 V
  Resistor1 : fl_lib/Electrical/Electrical Elements/Resistor  R=0.01 Ohm  i_specify=off  i_priority=High  i=0 A  i_nominal_specify=off  i_nominal_unit=A  i_nominal_value=1  v_specify=off  v_priority=High  v=0 V  v_nominal_specify=off  v_nominal_unit=V  v_nominal_value=1
  Resistor2 : fl_lib/Electrical/Electrical Elements/Resistor  R=0.005 Ohm  i_specify=off  i_priority=High  i=0 A  i_nominal_specify=off  i_nominal_unit=A  i_nominal_value=1  v_specify=off  v_priority=High  v=0 V  v_nominal_specify=off  v_nominal_unit=V  v_nominal_value=1
  + : PMIOPort  Side=Left
  - : PMIOPort  Port=2  Side=Right
  connections:
  Resistor2/LConn1 -- Capacitor/LConn1 -- Resistor1/RConn1
  DC Voltage Supply/RConn1 -- -/RConn1
  Resistor2/RConn1 -- +/RConn1 -- Capacitor/RConn1
  DC Voltage Supply/LConn1 -- Resistor1/LConn1

== system battery_pack_72v/Battery_pack/Mod14/Cell7 ==
  Capacitor : fl_lib/Electrical/Electrical Elements/Capacitor  c=5000 F  r=1e-6 Ohm  g=0 1/Ohm  i_specify=off  i_priority=High  i=0 A  i_nominal_specify=off  i_nominal_unit=A  i_nominal_value=1  v_specify=off  v_priority=High  v=0 V  v_nominal_specify=off  v_nominal_unit=V  v_nominal_value=1  vc_specify=on  vc_priority=High  vc=0 V  vc_nominal_specify=off  vc_nominal_unit=V  vc_nominal_value=1
  DC Voltage Supply : fl_lib/Electrical/Electrical Sources/DC Voltage Source  v0=3.6 V
  Resistor1 : fl_lib/Electrical/Electrical Elements/Resistor  R=0.01 Ohm  i_specify=off  i_priority=High  i=0 A  i_nominal_specify=off  i_nominal_unit=A  i_nominal_value=1  v_specify=off  v_priority=High  v=0 V  v_nominal_specify=off  v_nominal_unit=V  v_nominal_value=1
  Resistor2 : fl_lib/Electrical/Electrical Elements/Resistor  R=0.005 Ohm  i_specify=off  i_priority=High  i=0 A  i_nominal_specify=off  i_nominal_unit=A  i_nominal_value=1  v_specify=off  v_priority=High  v=0 V  v_nominal_specify=off  v_nominal_unit=V  v_nominal_value=1
  + : PMIOPort  Side=Left
  - : PMIOPort  Port=2  Side=Right
  connections:
  DC Voltage Supply/LConn1 -- Resistor1/LConn1
  Capacitor/RConn1 -- +/RConn1 -- Resistor2/RConn1
  DC Voltage Supply/RConn1 -- -/RConn1
  Resistor1/RConn1 -- Capacitor/LConn1 -- Resistor2/LConn1

== system battery_pack_72v/Battery_pack/Mod14/Cell8 ==
  Capacitor : fl_lib/Electrical/Electrical Elements/Capacitor  c=5000 F  r=1e-6 Ohm  g=0 1/Ohm  i_specify=off  i_priority=High  i=0 A  i_nominal_specify=off  i_nominal_unit=A  i_nominal_value=1  v_specify=off  v_priority=High  v=0 V  v_nominal_specify=off  v_nominal_unit=V  v_nominal_value=1  vc_specify=on  vc_priority=High  vc=0 V  vc_nominal_specify=off  vc_nominal_unit=V  vc_nominal_value=1
  DC Voltage Supply : fl_lib/Electrical/Electrical Sources/DC Voltage Source  v0=3.6 V
  Resistor1 : fl_lib/Electrical/Electrical Elements/Resistor  R=0.01 Ohm  i_specify=off  i_priority=High  i=0 A  i_nominal_specify=off  i_nominal_unit=A  i_nominal_value=1  v_specify=off  v_priority=High  v=0 V  v_nominal_specify=off  v_nominal_unit=V  v_nominal_value=1
  Resistor2 : fl_lib/Electrical/Electrical Elements/Resistor  R=0.005 Ohm  i_specify=off  i_priority=High  i=0 A  i_nominal_specify=off  i_nominal_unit=A  i_nominal_value=1  v_specify=off  v_priority=High  v=0 V  v_nominal_specify=off  v_nominal_unit=V  v_nominal_value=1
  + : PMIOPort  Side=Left
  - : PMIOPort  Port=2  Side=Right
  connections:
  Resistor2/LConn1 -- Capacitor/LConn1 -- Resistor1/RConn1
  DC Voltage Supply/RConn1 -- -/RConn1
  Resistor2/RConn1 -- +/RConn1 -- Capacitor/RConn1
  DC Voltage Supply/LConn1 -- Resistor1/LConn1

== system battery_pack_72v/Battery_pack/Mod14/Cell9 ==
  Capacitor : fl_lib/Electrical/Electrical Elements/Capacitor  c=5000 F  r=1e-6 Ohm  g=0 1/Ohm  i_specify=off  i_priority=High  i=0 A  i_nominal_specify=off  i_nominal_unit=A  i_nominal_value=1  v_specify=off  v_priority=High  v=0 V  v_nominal_specify=off  v_nominal_unit=V  v_nominal_value=1  vc_specify=on  vc_priority=High  vc=0 V  vc_nominal_specify=off  vc_nominal_unit=V  vc_nominal_value=1
  DC Voltage Supply : fl_lib/Electrical/Electrical Sources/DC Voltage Source  v0=3.6 V
  Resistor1 : fl_lib/Electrical/Electrical Elements/Resistor  R=0.01 Ohm  i_specify=off  i_priority=High  i=0 A  i_nominal_specify=off  i_nominal_unit=A  i_nominal_value=1  v_specify=off  v_priority=High  v=0 V  v_nominal_specify=off  v_nominal_unit=V  v_nominal_value=1
  Resistor2 : fl_lib/Electrical/Electrical Elements/Resistor  R=0.005 Ohm  i_specify=off  i_priority=High  i=0 A  i_nominal_specify=off  i_nominal_unit=A  i_nominal_value=1  v_specify=off  v_priority=High  v=0 V  v_nominal_specify=off  v_nominal_unit=V  v_nominal_value=1
  + : PMIOPort  Side=Left
  - : PMIOPort  Port=2  Side=Right
  connections:
  DC Voltage Supply/LConn1 -- Resistor1/LConn1
  Capacitor/RConn1 -- +/RConn1 -- Resistor2/RConn1
  DC Voltage Supply/RConn1 -- -/RConn1
  Resistor1/RConn1 -- Capacitor/LConn1 -- Resistor2/LConn1

== system battery_pack_72v/Battery_pack/Mod15/Cell1 ==
  Capacitor : fl_lib/Electrical/Electrical Elements/Capacitor  c=5000 F  r=1e-6 Ohm  g=0 1/Ohm  i_specify=off  i_priority=High  i=0 A  i_nominal_specify=off  i_nominal_unit=A  i_nominal_value=1  v_specify=off  v_priority=High  v=0 V  v_nominal_specify=off  v_nominal_unit=V  v_nominal_value=1  vc_specify=on  vc_priority=High  vc=0 V  vc_nominal_specify=off  vc_nominal_unit=V  vc_nominal_value=1
  DC Voltage Supply : fl_lib/Electrical/Electrical Sources/DC Voltage Source  v0=3.6 V
  Resistor1 : fl_lib/Electrical/Electrical Elements/Resistor  R=0.01 Ohm  i_specify=off  i_priority=High  i=0 A  i_nominal_specify=off  i_nominal_unit=A  i_nominal_value=1  v_specify=off  v_priority=High  v=0 V  v_nominal_specify=off  v_nominal_unit=V  v_nominal_value=1
  Resistor2 : fl_lib/Electrical/Electrical Elements/Resistor  R=0.005 Ohm  i_specify=off  i_priority=High  i=0 A  i_nominal_specify=off  i_nominal_unit=A  i_nominal_value=1  v_specify=off  v_priority=High  v=0 V  v_nominal_specify=off  v_nominal_unit=V  v_nominal_value=1
  + : PMIOPort  Side=Left
  - : PMIOPort  Port=2  Side=Right
  connections:
  Resistor2/LConn1 -- Capacitor/LConn1 -- Resistor1/RConn1
  DC Voltage Supply/RConn1 -- -/RConn1
  Resistor2/RConn1 -- +/RConn1 -- Capacitor/RConn1
  DC Voltage Supply/LConn1 -- Resistor1/LConn1

== system battery_pack_72v/Battery_pack/Mod15/Cell10 ==
  Capacitor : fl_lib/Electrical/Electrical Elements/Capacitor  c=5000 F  r=1e-6 Ohm  g=0 1/Ohm  i_specify=off  i_priority=High  i=0 A  i_nominal_specify=off  i_nominal_unit=A  i_nominal_value=1  v_specify=off  v_priority=High  v=0 V  v_nominal_specify=off  v_nominal_unit=V  v_nominal_value=1  vc_specify=on  vc_priority=High  vc=0 V  vc_nominal_specify=off  vc_nominal_unit=V  vc_nominal_value=1
  DC Voltage Supply : fl_lib/Electrical/Electrical Sources/DC Voltage Source  v0=3.6 V
  Resistor1 : fl_lib/Electrical/Electrical Elements/Resistor  R=0.01 Ohm  i_specify=off  i_priority=High  i=0 A  i_nominal_specify=off  i_nominal_unit=A  i_nominal_value=1  v_specify=off  v_priority=High  v=0 V  v_nominal_specify=off  v_nominal_unit=V  v_nominal_value=1
  Resistor2 : fl_lib/Electrical/Electrical Elements/Resistor  R=0.005 Ohm  i_specify=off  i_priority=High  i=0 A  i_nominal_specify=off  i_nominal_unit=A  i_nominal_value=1  v_specify=off  v_priority=High  v=0 V  v_nominal_specify=off  v_nominal_unit=V  v_nominal_value=1
  + : PMIOPort  Side=Left
  - : PMIOPort  Port=2  Side=Right
  connections:
  DC Voltage Supply/LConn1 -- Resistor1/LConn1
  Capacitor/RConn1 -- +/RConn1 -- Resistor2/RConn1
  DC Voltage Supply/RConn1 -- -/RConn1
  Resistor1/RConn1 -- Capacitor/LConn1 -- Resistor2/LConn1

== system battery_pack_72v/Battery_pack/Mod15/Cell11 ==
  Capacitor : fl_lib/Electrical/Electrical Elements/Capacitor  c=5000 F  r=1e-6 Ohm  g=0 1/Ohm  i_specify=off  i_priority=High  i=0 A  i_nominal_specify=off  i_nominal_unit=A  i_nominal_value=1  v_specify=off  v_priority=High  v=0 V  v_nominal_specify=off  v_nominal_unit=V  v_nominal_value=1  vc_specify=on  vc_priority=High  vc=0 V  vc_nominal_specify=off  vc_nominal_unit=V  vc_nominal_value=1
  DC Voltage Supply : fl_lib/Electrical/Electrical Sources/DC Voltage Source  v0=3.6 V
  Resistor1 : fl_lib/Electrical/Electrical Elements/Resistor  R=0.01 Ohm  i_specify=off  i_priority=High  i=0 A  i_nominal_specify=off  i_nominal_unit=A  i_nominal_value=1  v_specify=off  v_priority=High  v=0 V  v_nominal_specify=off  v_nominal_unit=V  v_nominal_value=1
  Resistor2 : fl_lib/Electrical/Electrical Elements/Resistor  R=0.005 Ohm  i_specify=off  i_priority=High  i=0 A  i_nominal_specify=off  i_nominal_unit=A  i_nominal_value=1  v_specify=off  v_priority=High  v=0 V  v_nominal_specify=off  v_nominal_unit=V  v_nominal_value=1
  + : PMIOPort  Side=Left
  - : PMIOPort  Port=2  Side=Right
  connections:
  Resistor2/LConn1 -- Capacitor/LConn1 -- Resistor1/RConn1
  DC Voltage Supply/RConn1 -- -/RConn1
  Resistor2/RConn1 -- +/RConn1 -- Capacitor/RConn1
  DC Voltage Supply/LConn1 -- Resistor1/LConn1

== system battery_pack_72v/Battery_pack/Mod15/Cell12 ==
  Capacitor : fl_lib/Electrical/Electrical Elements/Capacitor  c=5000 F  r=1e-6 Ohm  g=0 1/Ohm  i_specify=off  i_priority=High  i=0 A  i_nominal_specify=off  i_nominal_unit=A  i_nominal_value=1  v_specify=off  v_priority=High  v=0 V  v_nominal_specify=off  v_nominal_unit=V  v_nominal_value=1  vc_specify=on  vc_priority=High  vc=0 V  vc_nominal_specify=off  vc_nominal_unit=V  vc_nominal_value=1
  DC Voltage Supply : fl_lib/Electrical/Electrical Sources/DC Voltage Source  v0=3.6 V
  Resistor1 : fl_lib/Electrical/Electrical Elements/Resistor  R=0.01 Ohm  i_specify=off  i_priority=High  i=0 A  i_nominal_specify=off  i_nominal_unit=A  i_nominal_value=1  v_specify=off  v_priority=High  v=0 V  v_nominal_specify=off  v_nominal_unit=V  v_nominal_value=1
  Resistor2 : fl_lib/Electrical/Electrical Elements/Resistor  R=0.005 Ohm  i_specify=off  i_priority=High  i=0 A  i_nominal_specify=off  i_nominal_unit=A  i_nominal_value=1  v_specify=off  v_priority=High  v=0 V  v_nominal_specify=off  v_nominal_unit=V  v_nominal_value=1
  + : PMIOPort  Side=Left
  - : PMIOPort  Port=2  Side=Right
  connections:
  DC Voltage Supply/LConn1 -- Resistor1/LConn1
  Capacitor/RConn1 -- +/RConn1 -- Resistor2/RConn1
  DC Voltage Supply/RConn1 -- -/RConn1
  Resistor1/RConn1 -- Capacitor/LConn1 -- Resistor2/LConn1

== system battery_pack_72v/Battery_pack/Mod15/Cell15 ==
  Capacitor : fl_lib/Electrical/Electrical Elements/Capacitor  c=5000 F  r=1e-6 Ohm  g=0 1/Ohm  i_specify=off  i_priority=High  i=0 A  i_nominal_specify=off  i_nominal_unit=A  i_nominal_value=1  v_specify=off  v_priority=High  v=0 V  v_nominal_specify=off  v_nominal_unit=V  v_nominal_value=1  vc_specify=on  vc_priority=High  vc=0 V  vc_nominal_specify=off  vc_nominal_unit=V  vc_nominal_value=1
  DC Voltage Supply : fl_lib/Electrical/Electrical Sources/DC Voltage Source  v0=3.6 V
  Resistor1 : fl_lib/Electrical/Electrical Elements/Resistor  R=0.01 Ohm  i_specify=off  i_priority=High  i=0 A  i_nominal_specify=off  i_nominal_unit=A  i_nominal_value=1  v_specify=off  v_priority=High  v=0 V  v_nominal_specify=off  v_nominal_unit=V  v_nominal_value=1
  Resistor2 : fl_lib/Electrical/Electrical Elements/Resistor  R=0.005 Ohm  i_specify=off  i_priority=High  i=0 A  i_nominal_specify=off  i_nominal_unit=A  i_nominal_value=1  v_specify=off  v_priority=High  v=0 V  v_nominal_specify=off  v_nominal_unit=V  v_nominal_value=1
  + : PMIOPort  Side=Left
  - : PMIOPort  Port=2  Side=Right
  connections:
  Resistor2/LConn1 -- Capacitor/LConn1 -- Resistor1/RConn1
  DC Voltage Supply/RConn1 -- -/RConn1
  Resistor2/RConn1 -- +/RConn1 -- Capacitor/RConn1
  DC Voltage Supply/LConn1 -- Resistor1/LConn1

== system battery_pack_72v/Battery_pack/Mod15/Cell16 ==
  Capacitor : fl_lib/Electrical/Electrical Elements/Capacitor  c=5000 F  r=1e-6 Ohm  g=0 1/Ohm  i_specify=off  i_priority=High  i=0 A  i_nominal_specify=off  i_nominal_unit=A  i_nominal_value=1  v_specify=off  v_priority=High  v=0 V  v_nominal_specify=off  v_nominal_unit=V  v_nominal_value=1  vc_specify=on  vc_priority=High  vc=0 V  vc_nominal_specify=off  vc_nominal_unit=V  vc_nominal_value=1
  DC Voltage Supply : fl_lib/Electrical/Electrical Sources/DC Voltage Source  v0=3.6 V
  Resistor1 : fl_lib/Electrical/Electrical Elements/Resistor  R=0.01 Ohm  i_specify=off  i_priority=High  i=0 A  i_nominal_specify=off  i_nominal_unit=A  i_nominal_value=1  v_specify=off  v_priority=High  v=0 V  v_nominal_specify=off  v_nominal_unit=V  v_nominal_value=1
  Resistor2 : fl_lib/Electrical/Electrical Elements/Resistor  R=0.005 Ohm  i_specify=off  i_priority=High  i=0 A  i_nominal_specify=off  i_nominal_unit=A  i_nominal_value=1  v_specify=off  v_priority=High  v=0 V  v_nominal_specify=off  v_nominal_unit=V  v_nominal_value=1
  + : PMIOPort  Side=Left
  - : PMIOPort  Port=2  Side=Right
  connections:
  DC Voltage Supply/LConn1 -- Resistor1/LConn1
  Capacitor/RConn1 -- +/RConn1 -- Resistor2/RConn1
  DC Voltage Supply/RConn1 -- -/RConn1
  Resistor1/RConn1 -- Capacitor/LConn1 -- Resistor2/LConn1

== system battery_pack_72v/Battery_pack/Mod15/Cell17 ==
  Capacitor : fl_lib/Electrical/Electrical Elements/Capacitor  c=5000 F  r=1e-6 Ohm  g=0 1/Ohm  i_specify=off  i_priority=High  i=0 A  i_nominal_specify=off  i_nominal_unit=A  i_nominal_value=1  v_specify=off  v_priority=High  v=0 V  v_nominal_specify=off  v_nominal_unit=V  v_nominal_value=1  vc_specify=on  vc_priority=High  vc=0 V  vc_nominal_specify=off  vc_nominal_unit=V  vc_nominal_value=1
  DC Voltage Supply : fl_lib/Electrical/Electrical Sources/DC Voltage Source  v0=3.6 V
  Resistor1 : fl_lib/Electrical/Electrical Elements/Resistor  R=0.01 Ohm  i_specify=off  i_priority=High  i=0 A  i_nominal_specify=off  i_nominal_unit=A  i_nominal_value=1  v_specify=off  v_priority=High  v=0 V  v_nominal_specify=off  v_nominal_unit=V  v_nominal_value=1
  Resistor2 : fl_lib/Electrical/Electrical Elements/Resistor  R=0.005 Ohm  i_specify=off  i_priority=High  i=0 A  i_nominal_specify=off  i_nominal_unit=A  i_nominal_value=1  v_specify=off  v_priority=High  v=0 V  v_nominal_specify=off  v_nominal_unit=V  v_nominal_value=1
  + : PMIOPort  Side=Left
  - : PMIOPort  Port=2  Side=Right
  connections:
  Resistor2/LConn1 -- Capacitor/LConn1 -- Resistor1/RConn1
  DC Voltage Supply/RConn1 -- -/RConn1
  Resistor2/RConn1 -- +/RConn1 -- Capacitor/RConn1
  DC Voltage Supply/LConn1 -- Resistor1/LConn1
